simulink model "ass6_2_b1"  (R2023a)
settings: Solver=VariableStepAuto  StartTime=0.0  StopTime=10.0  RelTol=1e-3
settings Model: Creator=Taniya Baral  LastModifiedBy=Taniya Baral

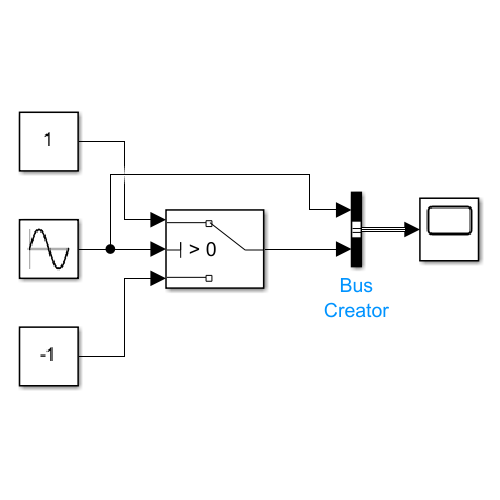
[thumbnail: Simulink's stored preview of the top-level diagram]
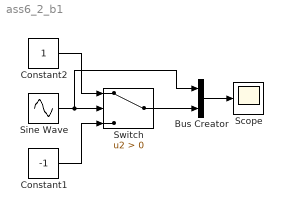
== system ass6_2_b1 ==
  Bus Creator : BusCreator  Inputs=2
  Constant1 : Constant  Value=-1
  Constant2 : Constant
  Scope : Scope
  Sine Wave : Sin  SampleTime=0
  Switch : Switch  Criteria=u2 > Threshold  SaturateOnIntegerOverflow=off  InputSameDT=off
  wires:
  Constant2/1 -> Switch/1
  Sine Wave/1 -> Bus Creator/1, Switch/2
  Constant1/1 -> Switch/3
  Switch/1 -> Bus Creator/2
  Bus Creator/1 -> Scope/1
